simulink model "soft_radio"  (Simulink 6.4)
settings: Solver=FixedStepDiscrete  StartTime=0.0  StopTime=inf  RelTol=1e-3
StartFcn:
  | soft_radio_init
values from neighbouring files (symbols this model uses):
  atten1 = 0.1    [SDR (2).m]
  atten2 = 0.78    [SDR (2).m]
  atten3 = 0.25    [SDR (2).m]
  delay1 = 55    [SDR (2).m]
  delay2inc = 2    [SDR (2).m]
  delay3inc = 2    [SDR (2).m]
  Fmod = Fs/4    (= 24000)    [SDR (2).m]
  freq_off = 10    [SDR (2).m]
  Fs = 96000    [SDR (2).m]
  pnoise = 0.0005    [SDR (2).m]
  Ts = 1/Fs    (= 1.04166666667e-05)    [SDR (2).m]
undefined symbols (not defined in the file or in its folder): get, gray, j
libraries: simulink x29, dspbuff3 x27, dspsigops x18, dspsrcs4 x10, dspstat3 x7, dspindex x6, dsparch4 x5, commsink2 x4, dspmtrx3 x4, dspsnks4 x3, dspxfrm3 x2, commnoisgen2 x1
CloseFcn:
  | rtwprivate ssgencode ModelCloseRequest soft_radio
settings Model: LastModifiedBy=isa  ProdHWDeviceType=32-bit Generic Real Time Simulator
settings DataIOCC: ExternalInput=a  LoadExternalInput=on  SaveFormat=Structure  SaveOutput=off  SaveTime=off
settings OptimizationCC: InlineParams=on  InlineInvariantSignals=on  EnforceIntegerDowncast=off  StateBitsets=on  DataBitsets=on  UseTempVars=on  EfficientFloat2IntCast=on
settings DebuggingCC: SignalResolutionControl=UseLocalSettings  InheritedTsInSrcMsg=none  IntegerOverflowMsg=none  StrictBusMsg=ErrorLevel1
settings HardwareCC: ProdHWDeviceType=32-bit Generic Real Time Simulator  TargetHWDeviceType=32-bit Generic
settings RTWCC: GenCodeOnly=on  ProcessScript=grt_make_rtw_hook

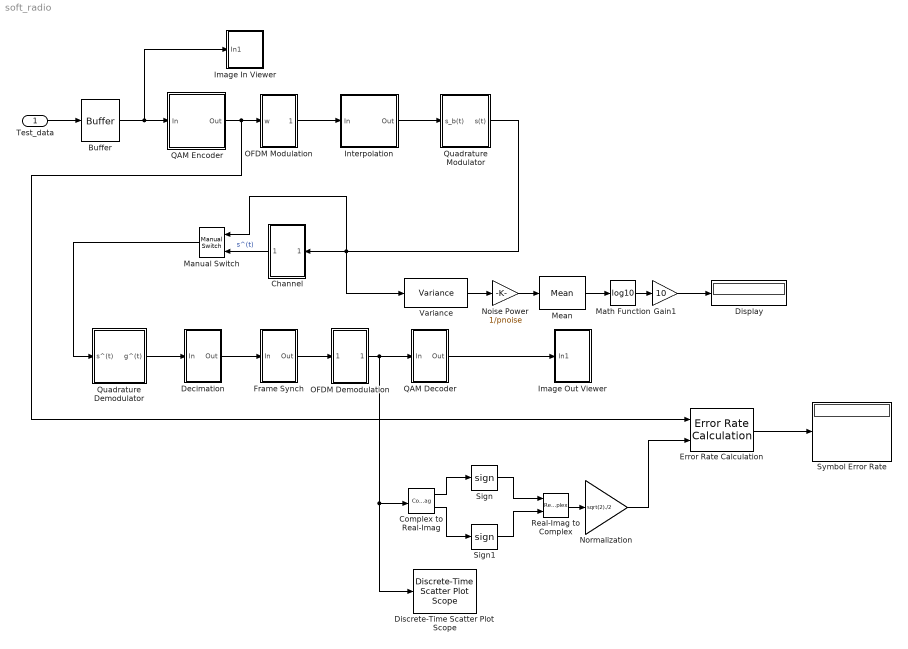
== system soft_radio ==
  Test_data : Inport  PortDimensions=1  SampleTime=1/(5*125)  DataType=uint8  Interpolate=off
  Buffer : dspbuff3/Buffer  N=256  V=0  ic=255
  Channel : Subsystem  Orientation=left
  Complex to Real-Imag : ComplexToRealImag
  Decimation : Subsystem
  Discrete-Time Scatter Plot Scope : commsink2/Discrete-Time Scatter Plot Scope  Tag=ScatterPlot  SystemSampleTime=-1  sampPerSymb=1  offsetEye=0  numTraces=40  numNewFrames=10  LineMarkers=.  LineColors=b  fading=on  render=on  AxisGrid=on  xMin=-1.87322652919263  xMax=1.91980304391689  yMin=-1.85318186191091  yMax=1.93984771119861  inphaseLabel=In-phase Amplitude  quadratureLabel=Quadrature Amplitude  openScopeAtSimStart=on  FrameNumber=off  FigPos=[360 138 560 560]  figTitle=Scatter Plot  numLinesMax=8  block_type_=scatter
  Display : Display
  Error Rate Calculation : commsink2/Error Rate Calculation  N=940  st_delay=0  cp_mode=Entire frame  subframe=[]  PMode=Port  WsName=ErrorVec  RsMode2=off  stop=off  numErr=1  maxBits=1
  Frame Synch : Subsystem
  Gain1 : Gain  Gain=10
  Image In Viewer : Subsystem
  Image Out Viewer : Subsystem
  "Interpolation " : Subsystem
  Manual Switch : simulink/Signal Routing/Manual Switch  Orientation=left  SystemSampleTime=-1  sw=1  action=0
  Math Function : Math  Operator=log10  SaturateOnIntegerOverflow=on
  Mean : dspstat3/Mean  DialogController=dspDDGCreate  DialogControllerArgs=DataTag10  run=on  reset_popup=None  roundingMode=Floor  overflowMode=off
  Noise Power : Gain  Gain=1/pnoise
  Normalization : Gain  Gain=sqrt(2)./2
  OFDM Demodulation : Subsystem
  OFDM Modulation : Subsystem
  QAM Decoder : Subsystem
  QAM Encoder : Subsystem
  Quadrature Demodulator : Subsystem
  Quadrature Modulator : Subsystem
  Real-Imag to Complex : RealImagToComplex
  Sign : Signum
  Sign1 : Signum
  Symbol Error Rate : Display
  Variance : dspstat3/Variance  DialogController=dspDDGCreate  DialogControllerArgs=DataTag15  run=off  reset_popup=None  roundingMode=Floor  overflowMode=off
  wires:
  Test_data/1 -> Buffer/1
  QAM Decoder/1(Out) -> Image Out Viewer/1(In1)
  Buffer/1 -> QAM Encoder/1(In), Image In Viewer/1(In1)
  OFDM Demodulation/1(w^) -> QAM Decoder/1(In), Discrete-Time Scatter Plot Scope/1, Complex to Real-Imag/1
  QAM Encoder/1(Out) -> OFDM Modulation/1(w), Error Rate Calculation/1
  OFDM Modulation/1(s_b(t)) -> "Interpolation "/1(In)
  "Interpolation "/1(Out) -> Quadrature Modulator/1(s_b(t))
  Quadrature Demodulator/1(g^(t)) -> Decimation/1(In)
  Decimation/1(Out) -> Frame Synch/1(In)
  Frame Synch/1(Out) -> OFDM Demodulation/1(g^(t))
  Quadrature Modulator/1(s(t)) -> Channel/1(s(t)), Manual Switch/1, Variance/1
  Channel/1(s^(t)) -> Manual Switch/2  "s^(t)"
  Manual Switch/1 -> Quadrature Demodulator/1(s^(t))
  Variance/1 -> Noise Power/1
  Noise Power/1 -> Mean/1
  Mean/1 -> Math Function/1
  Math Function/1 -> Gain1/1
  Gain1/1 -> Display/1
  Error Rate Calculation/1 -> Symbol Error Rate/1
  Complex to Real-Imag/1 -> Sign/1
  Complex to Real-Imag/2 -> Sign1/1
  Sign/1 -> Real-Imag to Complex/1
  Sign1/1 -> Real-Imag to Complex/2
  Real-Imag to Complex/1 -> Normalization/1
  Normalization/1 -> Error Rate Calculation/2

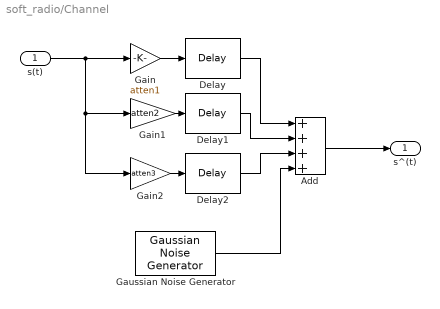
== system soft_radio/Channel ==
  s(t) : Inport
  Add : Sum  Inputs=++++  OutScaling=2^-10
  Delay : dspsigops/Delay  dly_unit=Samples  delay=delay1  ic_detail=off  dif_ic_for_ch=off  dif_ic_for_dly=off  ic=0  reset_popup=None
  Delay1 : dspsigops/Delay  dly_unit=Samples  delay=delay1+delay2inc  ic_detail=off  dif_ic_for_ch=off  dif_ic_for_dly=off  ic=0  reset_popup=None
  Delay2 : dspsigops/Delay  dly_unit=Samples  delay=delay1+delay3inc  ic_detail=off  dif_ic_for_ch=off  dif_ic_for_dly=off  ic=0  reset_popup=None
  Gain : Gain  Gain=atten1
  Gain1 : Gain  Gain=atten2
  Gain2 : Gain  Gain=atten3
  Gaussian Noise Generator : commnoisgen2/Gaussian Noise Generator  SystemSampleTime=-1  m=0  d=pnoise  s=noiseseed  Ts=-1  frameBased=on  sampPerFrame=96  orient=off  outDataType=double
  s^(t) : Outport
  wires:
  s(t)/1 -> Gain/1, Gain1/1, Gain2/1
  Gain/1 -> Delay/1
  Delay/1 -> Add/1
  Gain2/1 -> Delay2/1
  Gain1/1 -> Delay1/1
  Delay1/1 -> Add/2
  Delay2/1 -> Add/3
  Add/1 -> s^(t)/1
  Gaussian Noise Generator/1 -> Add/4

== system soft_radio/Decimation ==
  In : Inport
  Digital Filter Design : dsparch4/Digital Filter Design  SystemSampleTime=-1  mwdsp_browser_bugfix_var=off
  Digital Filter Design1 : dsparch4/Digital Filter Design  SystemSampleTime=-1  mwdsp_browser_bugfix_var=off
  Digital Filter Design2 : dsparch4/Digital Filter Design  SystemSampleTime=-1  mwdsp_browser_bugfix_var=off
  Downsample : dspsigops/Downsample  N=2  phase=0  ic=0  smode=Allow multirate  fmode=Maintain input frame size
  Downsample1 : dspsigops/Downsample  N=2  phase=0  ic=0  smode=Allow multirate  fmode=Maintain input frame size
  Downsample2 : dspsigops/Downsample  N=2  phase=0  ic=0  smode=Allow multirate  fmode=Maintain input frame size
  Out : Outport
  wires:
  Downsample/1 -> Out/1
  In/1 -> Digital Filter Design1/1
  Digital Filter Design1/1 -> Downsample1/1
  Downsample1/1 -> Digital Filter Design2/1
  Digital Filter Design2/1 -> Downsample2/1
  Downsample2/1 -> Digital Filter Design/1
  Digital Filter Design/1 -> Downsample/1

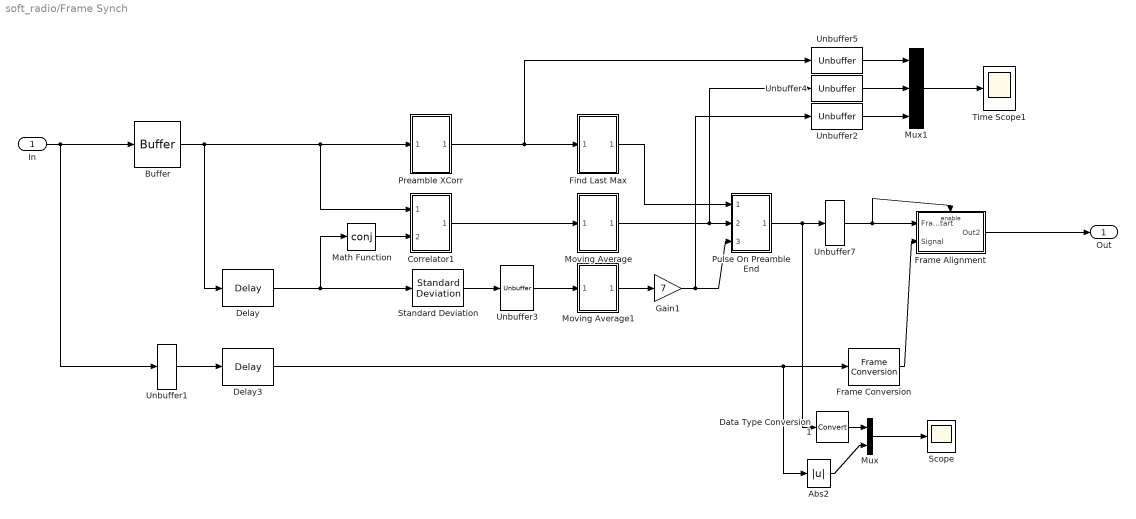
== system soft_radio/Frame Synch ==
  In : Inport
  Abs2 : Abs  SampleTime=-1  SaturateOnIntegerOverflow=off
  Buffer : dspbuff3/Buffer  N=161  V=160  ic=0
  Correlator1 : Subsystem
  Data Type Conversion1 : DataTypeConversion
  Delay : dspsigops/Delay  dly_unit=Frames  delay=161  ic_detail=off  dif_ic_for_ch=off  dif_ic_for_dly=off  ic=0  reset_popup=None
  Delay3 : dspsigops/Delay  dly_unit=Samples  delay=257-96  ic_detail=off  dif_ic_for_ch=off  dif_ic_for_dly=off  ic=0  reset_popup=None
  Find Last Max : Subsystem
  Frame Alignment : Subsystem  TreatAsAtomicUnit=on
  Frame Conversion : FrameConversion
  Gain1 : Gain  Gain=7
  Math Function : Math  Operator=conj  SaturateOnIntegerOverflow=on
  Moving Average : Subsystem
  Moving Average1 : Subsystem
  Mux : Mux  Inputs=2
  Mux1 : Mux  Inputs=3
  Preamble XCorr : Subsystem
  Pulse On Preamble End : Subsystem
  Scope : Scope
      settings: YMin=2.77556e-017  YMax=1  SaveName=frame_scope2  DataFormat=Array  MaxDataPoints=50000
  Standard Deviation : dspstat3/Standard Deviation  run=off  reset_popup=None
  Time Scope1 : Scope
      settings: TimeRange=3  YMin=5.55112e-017  YMax=2.1  DataFormat=Array  MaxDataPoints=50000
  Unbuffer{1..5,7} (6 alike) : dspbuff3/Unbuffer  ic=0
  Out : Outport
  wires:
  Buffer/1 -> Correlator1/1(In1), Preamble XCorr/1(In1), Delay/1
  In/1 -> Buffer/1, Unbuffer1/1
  Preamble XCorr/1(Out1) -> Find Last Max/1(In1), Unbuffer5/1
  Delay/1 -> Standard Deviation/1, Math Function/1
  Standard Deviation/1 -> Unbuffer3/1
  Unbuffer3/1 -> Moving Average1/1(In1)
  Moving Average/1(Out1) -> Pulse On Preamble End/2(In2), Unbuffer4/1
  Correlator1/1(Out1) -> Moving Average/1(In1)
  Moving Average1/1(Out1) -> Gain1/1
  Gain1/1 -> Pulse On Preamble End/3(In3), Unbuffer2/1
  Find Last Max/1(Out1) -> Pulse On Preamble End/1(In1)
  Pulse On Preamble End/1(Out1) -> Unbuffer7/1, Data Type Conversion1/1
  Delay3/1 -> Frame Conversion/1, Abs2/1
  Math Function/1 -> Correlator1/2(In2)
  Frame Conversion/1 -> Frame Alignment/2(Signal)
  Frame Alignment/1(Out2) -> Out/1
  Unbuffer7/1 -> Frame Alignment/1(Frame Start), Frame Alignment/Enable
  Abs2/1 -> Mux/2
  Mux/1 -> Scope/1
  Data Type Conversion1/1 -> Mux/1
  Mux1/1 -> Time Scope1/1
  Unbuffer2/1 -> Mux1/3
  Unbuffer4/1 -> Mux1/2
  Unbuffer5/1 -> Mux1/1
  Unbuffer1/1 -> Delay3/1

== system soft_radio/Image In Viewer ==
  In1 : Inport  Orientation=down
  Delay Line : dspbuff3/Delay Line  siz=256  ic=0  directfeed=off
  Matrix Viewer : dspsnks4/Matrix Viewer  DialogController=dspdialog.MatrixViewer  DialogControllerArgs=DataTag6  ImageParams=off  CMapStr=gray(256)  AxisColorbar=on  AxisParams=off  AxisOrigin=Upper left corner  XLabel=X-axis  YLabel=Y-axis  ZLabel=Z-axis  FigPos=get(0,'defaultfigureposition')  AxisZoom=off
      settings: YMin=0  YMax=255
  Transpose : dspmtrx3/Transpose  SystemSampleTime=-1  Hermitian=off  overflowFlag=on
  Transpose2 : dspmtrx3/Transpose  SystemSampleTime=-1  Hermitian=off  overflowFlag=on
  wires:
  In1/1 -> Transpose/1
  Transpose2/1 -> Matrix Viewer/1
  Delay Line/1 -> Transpose2/1
  Transpose/1 -> Delay Line/1

== system soft_radio/Image Out Viewer ==
  In1 : Inport  Orientation=down
  Delay Line : dspbuff3/Delay Line  siz=256  ic=0  directfeed=off
  Matrix Viewer : dspsnks4/Matrix Viewer  DialogController=dspdialog.MatrixViewer  DialogControllerArgs=DataTag7  ImageParams=off  CMapStr=gray(256)  AxisColorbar=on  AxisParams=off  AxisOrigin=Upper left corner  XLabel=X-axis  YLabel=Y-axis  ZLabel=Z-axis  FigPos=get(0,'defaultfigureposition')  AxisZoom=off
      settings: YMin=0  YMax=255
  Transpose : dspmtrx3/Transpose  SystemSampleTime=-1  Hermitian=off  overflowFlag=on
  Transpose2 : dspmtrx3/Transpose  SystemSampleTime=-1  Hermitian=off  overflowFlag=on
  wires:
  Transpose/1 -> Delay Line/1
  Delay Line/1 -> Transpose2/1
  Transpose2/1 -> Matrix Viewer/1
  In1/1 -> Transpose/1

== system soft_radio/Interpolation  ==
  In : Inport
  Initial Upsampling Filter : dsparch4/Digital Filter Design  SystemSampleTime=-1  mwdsp_browser_bugfix_var=off
  Second Upsample : dspsigops/Upsample  N=4  phase=0  ic=0  mode=Maintain input frame size
  Second Upsampling Filter : dsparch4/Digital Filter Design  SystemSampleTime=-1  mwdsp_browser_bugfix_var=off
  Upsample : dspsigops/Upsample  N=2  phase=0  ic=0  mode=Maintain input frame size
  Upsampling Amplitude Correction : Gain  Gain=8
  Out : Outport
  wires:
  Initial Upsampling Filter/1 -> Second Upsample/1
  Upsample/1 -> Initial Upsampling Filter/1
  Second Upsample/1 -> Second Upsampling Filter/1
  In/1 -> Upsample/1
  Second Upsampling Filter/1 -> Upsampling Amplitude Correction/1
  Upsampling Amplitude Correction/1 -> Out/1

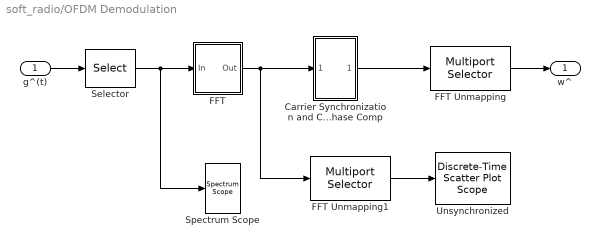
== system soft_radio/OFDM Demodulation ==
  g^(t) : Inport
  Carrier Synchronization and Channel Phase Comp : Subsystem
  FFT : Subsystem
  FFT Unmapping : dspindex/Multiport Selector  rowsOrCols=Rows  idxCellArray={[2, 3, 4, 5, 61, 62, 63, 64, 6, 7, 59, 60, 9, 10, 11, 12, 54, 55, 56, 57]}  idxErrMode=Clip Index
  FFT Unmapping1 : dspindex/Multiport Selector  rowsOrCols=Rows  idxCellArray={[2, 3, 4, 5, 61, 62, 63, 64, 6, 7, 59, 60, 9, 10, 11, 12, 54, 55, 56, 57]}  idxErrMode=Clip Index
  Selector : Selector  Elements=[25:88]  InputPortWidth=96
  Spectrum Scope : dspsnks4/Spectrum Scope  DialogController=dspdialog.SpectrumScope  DialogControllerArgs=DataTag13  SystemSampleTime=-1  ScopeProperties=on  Domain=Frequency  HorizSpan=1  UseBuffer=on  BufferSize=64  Overlap=0  inpFftLenInherit=off  FFTlength=128  numAvg=2  DisplayProperties=off  AxisGrid=on  Memory=off  FrameNumber=on  AxisLegend=off  AxisZoom=off  OpenScopeAtSimStart=on  OpenScopeImmediately=off  FigPos=get(0,'defaultfigureposition')  AxisProperties=off  XUnits=Hertz  XRange=[-Fs/2...Fs/2]  InheritXIncr=on  XIncr=1.0  XLabel=Samples  YUnits=dB  YLabel=Magnitude-squared, dB  LineProperties=off  wintypeSpecScope=Hann  RsSpecScope=50  betaSpecScope=5  winsampSpecScope=Periodic
      settings: YMin=-120.845322888998  YMax=-11.741242369477
  Unsynchronized : commsink2/Discrete-Time Scatter Plot Scope  Tag=ScatterPlot  SystemSampleTime=-1  sampPerSymb=1  offsetEye=0  numTraces=40  numNewFrames=10  LineMarkers=.  LineColors=b  fading=on  render=on  AxisGrid=on  xMin=-1.88995217282586  xMax=1.90933368918377  yMin=-1.88734763336516  yMax=1.91193822864447  inphaseLabel=In-phase Amplitude  quadratureLabel=Quadrature Amplitude  openScopeAtSimStart=on  FrameNumber=off  FigPos=[360 138 560 560]  figTitle=Scatter Plot  numLinesMax=8  block_type_=scatter
  w^ : Outport
  wires:
  g^(t)/1 -> Selector/1
  FFT Unmapping/1 -> w^/1
  Selector/1 -> FFT/1(In), Spectrum Scope/1
  FFT/1(Out) -> FFT Unmapping1/1, Carrier Synchronization and Channel Phase Comp/1(s(f))
  FFT Unmapping1/1 -> Unsynchronized/1
  Carrier Synchronization and Channel Phase Comp/1(s^(f)) -> FFT Unmapping/1

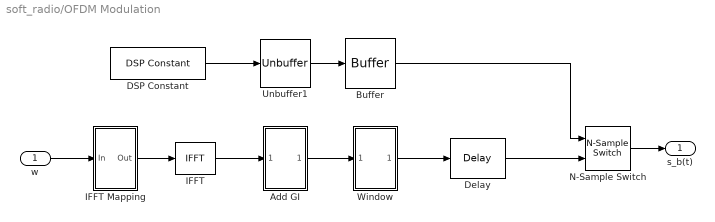
== system soft_radio/OFDM Modulation ==
  w : Inport
  Add GI : Subsystem
  Buffer : dspbuff3/Buffer  N=96  V=0  ic=0
  DSP Constant : dspsrcs4/DSP Constant  SystemSampleTime=-1  Value=preamble_whole'  SampleMode=Discrete  discreteOutput=Frame-based  continuousOutput=Sample-based  sampTime=-1  framePeriod=-1  dataType=Inherit from 'Constant value'  isSigned=on  wordLen=16  udDataType=sfix(16)  fracBitsMode=Best precision  numFracBits=15  InterpretAs1D=-inf  Ts=-inf  FramebasedOutput=-inf
  Delay : dspsigops/Delay  dly_unit=Frames  delay=39  ic_detail=off  dif_ic_for_ch=off  dif_ic_for_dly=off  ic=0  reset_popup=None
  IFFT : dspxfrm3/IFFT  DialogController=dspDDGCreate  DialogControllerArgs=DataTag14  CompMethod=Table lookup  TableOpt=Speed  BitRevOrder=off  cs_in=off  SkipNorm=off  mode=Complex  roundingMode=Floor  overflowMode=off
  IFFT Mapping : Subsystem
  N-Sample Switch : dspswit3/N-Sample Switch  SystemSampleTime=-1  N=39  reset=off  TriggerType=Rising edge  Ts=-1
  Unbuffer1 : dspbuff3/Unbuffer  ic=0
  Window : Subsystem
  s_b(t) : Outport
  wires:
  IFFT Mapping/1(Out) -> IFFT/1
  w/1 -> IFFT Mapping/1(In)
  IFFT/1 -> Add GI/1(In1)
  Add GI/1(Out1) -> Window/1(In1)
  Window/1(Out1) -> Delay/1
  N-Sample Switch/1 -> s_b(t)/1
  Buffer/1 -> N-Sample Switch/1
  DSP Constant/1 -> Unbuffer1/1
  Unbuffer1/1 -> Buffer/1
  Delay/1 -> N-Sample Switch/2

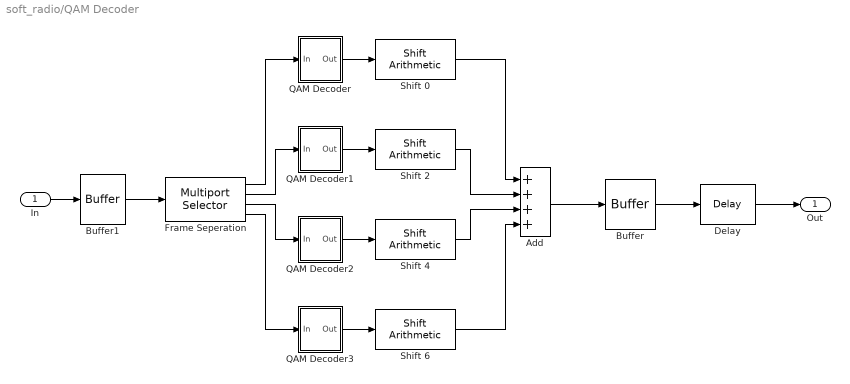
== system soft_radio/QAM Decoder ==
  In : Inport
  Add : Sum  Inputs=++++  OutScaling=2^-10
  Buffer : dspbuff3/Buffer  N=256  V=0  ic=0
  Buffer1 : dspbuff3/Buffer  N=4  V=0  ic=0
  Delay : dspsigops/Delay  dly_unit=Samples  delay=11  ic_detail=off  dif_ic_for_ch=off  dif_ic_for_dly=off  ic=0  reset_popup=None
  Frame Seperation : dspindex/Multiport Selector  rowsOrCols=Rows  idxCellArray={1,2,3,4}  idxErrMode=Clip Index
  QAM Decoder : Subsystem
  QAM Decoder1 : Subsystem
  QAM Decoder2 : Subsystem
  QAM Decoder3 : Subsystem
  Shift 0 : simulink/Logic and Bit Operations/Shift Arithmetic  SystemSampleTime=-1  nBitShiftRight=0  nBinPtShiftRight=0
  Shift 2 : simulink/Logic and Bit Operations/Shift Arithmetic  SystemSampleTime=-1  nBitShiftRight=-2  nBinPtShiftRight=0
  Shift 4 : simulink/Logic and Bit Operations/Shift Arithmetic  SystemSampleTime=-1  nBitShiftRight=-4  nBinPtShiftRight=0
  Shift 6 : simulink/Logic and Bit Operations/Shift Arithmetic  SystemSampleTime=-1  nBitShiftRight=-6  nBinPtShiftRight=0
  Out : Outport
  wires:
  Frame Seperation/1 -> QAM Decoder/1(In)
  QAM Decoder/1(Out) -> Shift 0/1
  Frame Seperation/2 -> QAM Decoder1/1(In)
  Frame Seperation/3 -> QAM Decoder2/1(In)
  Frame Seperation/4 -> QAM Decoder3/1(In)
  QAM Decoder1/1(Out) -> Shift 2/1
  QAM Decoder2/1(Out) -> Shift 4/1
  QAM Decoder3/1(Out) -> Shift 6/1
  Shift 0/1 -> Add/1
  Shift 2/1 -> Add/2
  Shift 4/1 -> Add/3
  Shift 6/1 -> Add/4
  Add/1 -> Buffer/1
  In/1 -> Buffer1/1
  Buffer/1 -> Delay/1
  Delay/1 -> Out/1
  Buffer1/1 -> Frame Seperation/1

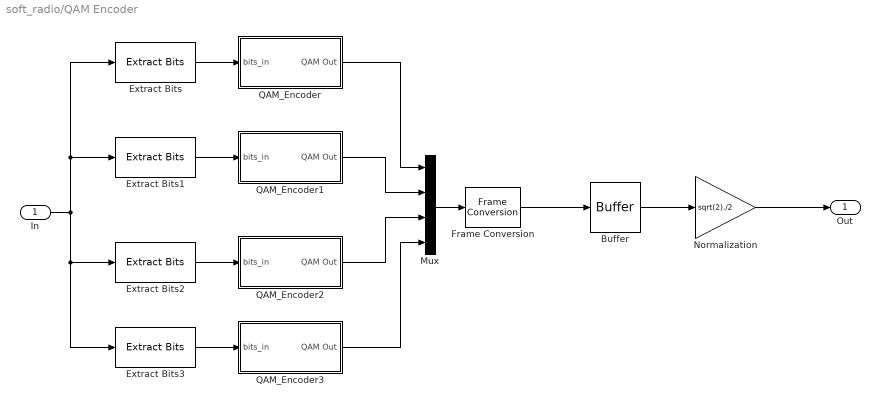
== system soft_radio/QAM Encoder ==
  In : Inport
  Buffer : dspbuff3/Buffer  N=20  V=0  ic=-1-j
  Extract Bits : simulink/Logic and Bit Operations/Extract Bits  SystemSampleTime=-1  bitsToExtract=Range of bits  numBits=2  bitIdxRange=[0 1]  outScalingMode=Treat bit field as an integer
  Extract Bits1 : simulink/Logic and Bit Operations/Extract Bits  SystemSampleTime=-1  bitsToExtract=Range of bits  numBits=2  bitIdxRange=[2 3]  outScalingMode=Treat bit field as an integer
  Extract Bits2 : simulink/Logic and Bit Operations/Extract Bits  SystemSampleTime=-1  bitsToExtract=Range of bits  numBits=2  bitIdxRange=[4 5]  outScalingMode=Treat bit field as an integer
  Extract Bits3 : simulink/Logic and Bit Operations/Extract Bits  SystemSampleTime=-1  bitsToExtract=Range of bits  numBits=2  bitIdxRange=[6 7]  outScalingMode=Treat bit field as an integer
  Frame Conversion : FrameConversion
  Mux : Mux
  Normalization : Gain  Gain=sqrt(2)./2
  QAM_Encoder : Subsystem
  QAM_Encoder1 : Subsystem
  QAM_Encoder2 : Subsystem
  QAM_Encoder3 : Subsystem
  Out : Outport
  wires:
  In/1 -> Extract Bits1/1, Extract Bits/1, Extract Bits2/1, Extract Bits3/1
  Extract Bits/1 -> QAM_Encoder/1(bits_in)
  Extract Bits1/1 -> QAM_Encoder1/1(bits_in)
  Extract Bits2/1 -> QAM_Encoder2/1(bits_in)
  Extract Bits3/1 -> QAM_Encoder3/1(bits_in)
  QAM_Encoder/1(QAM Out) -> Mux/1
  QAM_Encoder1/1(QAM Out) -> Mux/2
  QAM_Encoder2/1(QAM Out) -> Mux/3
  QAM_Encoder3/1(QAM Out) -> Mux/4
  Mux/1 -> Frame Conversion/1
  Frame Conversion/1 -> Buffer/1
  Buffer/1 -> Normalization/1
  Normalization/1 -> Out/1

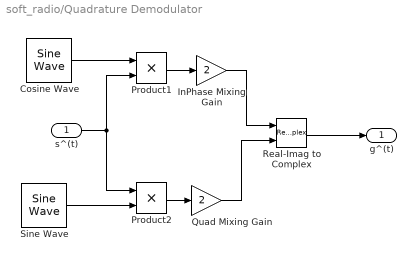
== system soft_radio/Quadrature Demodulator ==
  s^(t) : Inport
  Cosine Wave : dspsrcs4/Sine Wave  Amplitude=1  Frequency=Fmod+freq_off  Phase=pi/2  SampleMode=Discrete  OutComplex=Real  CompMethod=Trigonometric fcn  TableSize=Speed  SampleTime=Ts  SamplesPerFrame=96  dataType=double  wordLen=16  udDataType=sfix(16)  fracBitsMode=Best precision  numFracBits=15  ResetState=Restart at time zero
  InPhase Mixing Gain : Gain  Gain=2
  Product1 : Product  RndMeth=Zero
  Product2 : Product  RndMeth=Zero
  Quad Mixing Gain : Gain  Gain=2
  Real-Imag to Complex : RealImagToComplex
  Sine Wave : dspsrcs4/Sine Wave  Amplitude=1  Frequency=Fmod+freq_off  Phase=0  SampleMode=Discrete  OutComplex=Real  CompMethod=Trigonometric fcn  TableSize=Speed  SampleTime=Ts  SamplesPerFrame=96  dataType=double  wordLen=16  udDataType=sfix(16)  fracBitsMode=Best precision  numFracBits=15  ResetState=Restart at time zero
  g^(t) : Outport
  wires:
  s^(t)/1 -> Product1/2, Product2/1
  Cosine Wave/1 -> Product1/1
  Sine Wave/1 -> Product2/2
  Product1/1 -> InPhase Mixing Gain/1
  Product2/1 -> Quad Mixing Gain/1
  Quad Mixing Gain/1 -> Real-Imag to Complex/2
  InPhase Mixing Gain/1 -> Real-Imag to Complex/1
  Real-Imag to Complex/1 -> g^(t)/1

== system soft_radio/Quadrature Modulator ==
  s_b(t) : Inport
  Add : Sum  OutScaling=2^-10
  Complex to Real-Imag : ComplexToRealImag
  Cosine Wave : dspsrcs4/Sine Wave  Amplitude=1  Frequency=Fmod  Phase=pi/2  SampleMode=Discrete  OutComplex=Real  CompMethod=Trigonometric fcn  TableSize=Speed  SampleTime=Ts  SamplesPerFrame=96  dataType=double  wordLen=16  udDataType=sfix(16)  fracBitsMode=Best precision  numFracBits=15  ResetState=Restart at time zero
  Product : Product  RndMeth=Zero
  Product2 : Product  RndMeth=Zero
  Sine Wave : dspsrcs4/Sine Wave  Amplitude=1  Frequency=Fmod  Phase=0  SampleMode=Discrete  OutComplex=Real  CompMethod=Trigonometric fcn  TableSize=Speed  SampleTime=Ts  SamplesPerFrame=96  dataType=double  wordLen=16  udDataType=sfix(16)  fracBitsMode=Best precision  numFracBits=15  ResetState=Restart at time zero
  s(t) : Outport
  wires:
  Add/1 -> s(t)/1
  Product/1 -> Add/1
  Product2/1 -> Add/2
  Cosine Wave/1 -> Product/1
  s_b(t)/1 -> Complex to Real-Imag/1
  Complex to Real-Imag/2 -> Product2/1
  Complex to Real-Imag/1 -> Product/2
  Sine Wave/1 -> Product2/2

== system soft_radio/Frame Synch/Correlator1 ==
  In1 : Inport
  In2 : Inport  Port=2
  Abs2 : Abs  SampleTime=-1  SaturateOnIntegerOverflow=off
  Product1 : Product  RndMeth=Zero
  Sum of Elements1 : Sum  Inputs=+  OutScaling=2^-10
  Out1 : Outport
  wires:
  Product1/1 -> Sum of Elements1/1
  Sum of Elements1/1 -> Abs2/1
  In1/1 -> Product1/1
  In2/1 -> Product1/2
  Abs2/1 -> Out1/1

== system soft_radio/Frame Synch/Find Last Max ==
  In1 : Inport
  Compare To Constant : simulink/Logic and Bit Operations/Compare To Constant  SystemSampleTime=-1  relop===  const=64  LogicOutDataTypeMode=uint8  ZeroCross=off
  Delay Line1 : dspbuff3/Delay Line  siz=64  ic=0  directfeed=off
  Maximum : dspstat3/Maximum  DialogController=dspDDGCreate  DialogControllerArgs=DataTag3  fcn=Index  reset=None  roundingMode=Floor  overflowMode=off
  Out1 : Outport
  wires:
  Delay Line1/1 -> Maximum/1
  Maximum/1 -> Compare To Constant/1
  In1/1 -> Delay Line1/1
  Compare To Constant/1 -> Out1/1

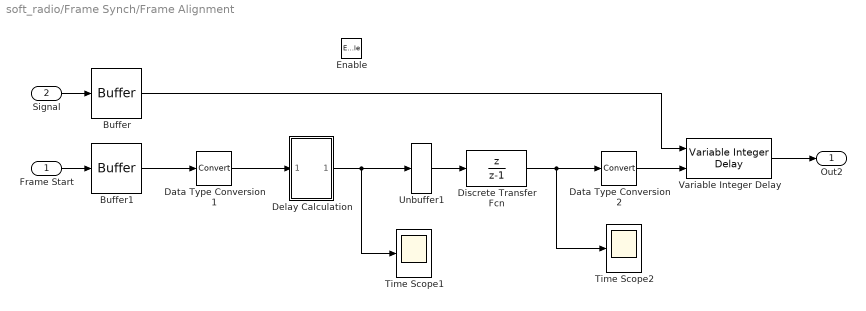
== system soft_radio/Frame Synch/Frame Alignment ==
  Frame Start : Inport
  Signal : Inport  Port=2
      settings: SignalType=complex
  Enable : EnablePort  StatesWhenEnabling=reset
  Buffer : dspbuff3/Buffer  N=96  V=0  ic=0
  Buffer1 : dspbuff3/Buffer  N=96  V=0  ic=0
  Data Type Conversion1 : DataTypeConversion
  Data Type Conversion2 : DataTypeConversion
  Delay Calculation : Subsystem
  Discrete Transfer Fcn : DiscreteTransferFcn  Numerator=[1 0]  Denominator=[1 -1]  SampleTime=-1
  Time Scope1 : Scope
      settings: YMax=10  SaveName=ScopeData3  DataFormat=Structure
  Time Scope2 : Scope
      settings: YMin=0  YMax=70  SaveName=ScopeData2  DataFormat=Structure
  Unbuffer1 : dspbuff3/Unbuffer  ic=0
  Variable Integer Delay : dspsigops/Variable Integer Delay  dmax=100  ic=0
  Out2 : Outport  InitialOutput=[-2*ones(64,0)]
  wires:
  Signal/1 -> Buffer/1
  Frame Start/1 -> Buffer1/1
  Buffer1/1 -> Data Type Conversion1/1
  Delay Calculation/1(Out1) -> Time Scope1/1, Unbuffer1/1
  Variable Integer Delay/1 -> Out2/1
  Discrete Transfer Fcn/1 -> Data Type Conversion2/1, Time Scope2/1
  Data Type Conversion1/1 -> Delay Calculation/1(In1)
  Buffer/1 -> Variable Integer Delay/1
  Unbuffer1/1 -> Discrete Transfer Fcn/1
  Data Type Conversion2/1 -> Variable Integer Delay/2

== system soft_radio/Frame Synch/Moving Average ==
  In1 : Inport
  Delay Line : dspbuff3/Delay Line  siz=128  ic=0  directfeed=off
  Mean : dspstat3/Mean  DialogController=dspDDGCreate  DialogControllerArgs=DataTag4  run=off  reset_popup=None  roundingMode=Floor  overflowMode=off
  Out1 : Outport
  wires:
  Delay Line/1 -> Mean/1
  In1/1 -> Delay Line/1
  Mean/1 -> Out1/1

== system soft_radio/Frame Synch/Moving Average1 ==
  In1 : Inport
  Delay Line2 : dspbuff3/Delay Line  siz=64  ic=0  directfeed=off
  Mean1 : dspstat3/Mean  DialogController=dspDDGCreate  DialogControllerArgs=DataTag5  run=off  reset_popup=None  roundingMode=Floor  overflowMode=off
  Out1 : Outport
  wires:
  Delay Line2/1 -> Mean1/1
  In1/1 -> Delay Line2/1
  Mean1/1 -> Out1/1

== system soft_radio/Frame Synch/Preamble XCorr ==
  In1 : Inport  Orientation=down
  Correlator : Subsystem
  Math Function1 : Math  Operator=conj  SaturateOnIntegerOverflow=on
  Short Sequence : dspsrcs4/DSP Constant  SystemSampleTime=-1  Value=short_seq_r'  SampleMode=Discrete  discreteOutput=Frame-based  continuousOutput=Sample-based  sampTime=1/(96e3)  framePeriod=-1  dataType=Inherit from 'Constant value'  isSigned=on  wordLen=16  udDataType=sfix(16)  fracBitsMode=Best precision  numFracBits=15  InterpretAs1D=-inf  Ts=-inf  FramebasedOutput=-inf
  Out1 : Outport
  wires:
  Short Sequence/1 -> Math Function1/1
  Math Function1/1 -> Correlator/1(In1)
  In1/1 -> Correlator/2(In2)
  Correlator/1(Out1) -> Out1/1

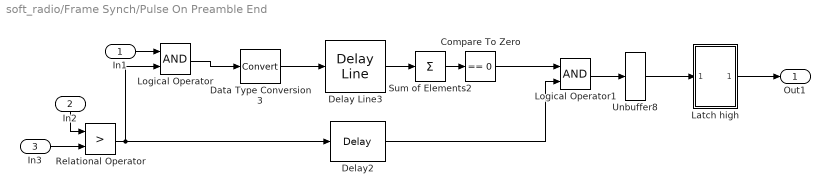
== system soft_radio/Frame Synch/Pulse On Preamble End ==
  In1 : Inport
  In2 : Inport  Orientation=down  Port=2
  In3 : Inport  Port=3
  Compare To Zero : simulink/Logic and Bit Operations/Compare To Zero  SystemSampleTime=-1  relop===  LogicOutDataTypeMode=uint8  ZeroCross=off
  Data Type Conversion3 : DataTypeConversion
  Delay Line3 : dspbuff3/Delay Line  siz=256  ic=0  directfeed=off
  Delay2 : dspsigops/Delay  dly_unit=Samples  delay=256  ic_detail=off  dif_ic_for_ch=off  dif_ic_for_dly=off  ic=0  reset_popup=None
  Latch high : Subsystem
  Logical Operator : Logic  AllPortsSameDT=off  OutDataTypeMode=Boolean
  Logical Operator1 : Logic  AllPortsSameDT=off  OutDataTypeMode=Boolean
  Relational Operator : RelationalOperator  Operator=>  LogicOutDataTypeMode=Boolean
  Sum of Elements2 : Sum  Inputs=+  OutScaling=2^-10
  Unbuffer8 : dspbuff3/Unbuffer  ic=0
  Out1 : Outport
  wires:
  Relational Operator/1 -> Logical Operator/2, Delay2/1
  Logical Operator/1 -> Data Type Conversion3/1
  Data Type Conversion3/1 -> Delay Line3/1
  Delay Line3/1 -> Sum of Elements2/1
  Sum of Elements2/1 -> Compare To Zero/1
  Compare To Zero/1 -> Logical Operator1/1
  Delay2/1 -> Logical Operator1/2
  In2/1 -> Relational Operator/1
  In3/1 -> Relational Operator/2
  In1/1 -> Logical Operator/1
  Logical Operator1/1 -> Unbuffer8/1
  Latch high/1(Out1) -> Out1/1
  Unbuffer8/1 -> Latch high/1(In1)

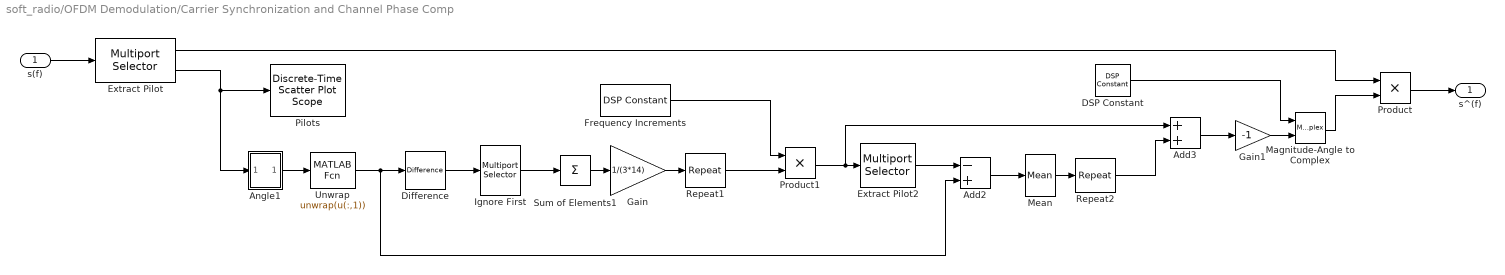
== system soft_radio/OFDM Demodulation/Carrier Synchronization and Channel Phase Comp ==
  s(f) : Inport
  Add2 : Sum  Inputs=-+  OutScaling=2^-10
  Add3 : Sum  OutScaling=2^-10
  Angle1 : Subsystem
  DSP Constant : dspsrcs4/DSP Constant  SystemSampleTime=-1  Value=1  SampleMode=Discrete  discreteOutput=Sample-based  continuousOutput=Sample-based  sampTime=-1  framePeriod=2  dataType=Inherit from 'Constant value'  isSigned=on  wordLen=16  udDataType=sfix(16)  fracBitsMode=Best precision  numFracBits=15  InterpretAs1D=-inf  Ts=-inf  FramebasedOutput=-inf
  Difference : simulink/Discrete/Difference  SystemSampleTime=-1  ICPrevInput=0.0  OutDataType=sfix(16)  OutScaling=2^-10  DoSatur=off
  Extract Pilot : dspindex/Multiport Selector  rowsOrCols=Rows  idxCellArray={[1:64],[44, 58, 8, 22]}  idxErrMode=Clip Index
  Extract Pilot2 : dspindex/Multiport Selector  rowsOrCols=Rows  idxCellArray={[44, 58, 8, 22]}  idxErrMode=Clip Index
  Frequency Increments : dspsrcs4/DSP Constant  SystemSampleTime=-1  Value=[32:63 0:31]'  SampleMode=Discrete  discreteOutput=Sample-based  continuousOutput=Sample-based  sampTime=-1  framePeriod=2  dataType=Inherit from 'Constant value'  isSigned=on  wordLen=16  udDataType=sfix(16)  fracBitsMode=Best precision  numFracBits=15  InterpretAs1D=-inf  Ts=-inf  FramebasedOutput=-inf
  Gain : Gain  Gain=1/(3*14)
  Gain1 : Gain  Gain=-1
  Ignore First : dspindex/Multiport Selector  rowsOrCols=Rows  idxCellArray={[2:4]}  idxErrMode=Clip Index
  Magnitude-Angle to Complex : MagnitudeAngleToComplex
  Mean : dspstat3/Mean  DialogController=dspDDGCreate  DialogControllerArgs=DataTag11  run=off  reset_popup=None  roundingMode=Floor  overflowMode=off
  Pilots : commsink2/Discrete-Time Scatter Plot Scope  Tag=ScatterPlot  SystemSampleTime=-1  sampPerSymb=1  offsetEye=0  numTraces=40  numNewFrames=10  LineMarkers=.  LineColors=b  fading=on  render=on  AxisGrid=on  xMin=-1.3  xMax=1.3  yMin=-1.3  yMax=1.3  inphaseLabel=In-phase Amplitude  quadratureLabel=Quadrature Amplitude  openScopeAtSimStart=off  FrameNumber=off  FigPos=[360 138 560 560]  figTitle=Scatter Plot  numLinesMax=8  block_type_=scatter
  Product : Product  RndMeth=Zero
  Product1 : Product  RndMeth=Zero
  Repeat1 : dspsigops/Repeat  N=64  ic=0  mode=Maintain input frame rate
  Repeat2 : dspsigops/Repeat  N=64  ic=0  mode=Maintain input frame rate
  Sum of Elements1 : Sum  Inputs=+  OutScaling=2^-10
  Unwrap : MATLABFcn  MATLABFcn=unwrap(u(:,1))  Output1D=off
  s^(f) : Outport
  wires:
  DSP Constant/1 -> Magnitude-Angle to Complex/1
  Magnitude-Angle to Complex/1 -> Product/2
  Product/1 -> s^(f)/1
  Extract Pilot/2 -> Angle1/1(In), Pilots/1
  s(f)/1 -> Extract Pilot/1
  Extract Pilot/1 -> Product/1
  Difference/1 -> Ignore First/1
  Sum of Elements1/1 -> Gain/1
  Gain/1 -> Repeat1/1
  Angle1/1(Out) -> Unwrap/1
  Unwrap/1 -> Difference/1, Add2/2
  Ignore First/1 -> Sum of Elements1/1
  Frequency Increments/1 -> Product1/1
  Repeat1/1 -> Product1/2
  Product1/1 -> Extract Pilot2/1, Add3/1
  Extract Pilot2/1 -> Add2/1
  Add2/1 -> Mean/1
  Mean/1 -> Repeat2/1
  Repeat2/1 -> Add3/2
  Add3/1 -> Gain1/1
  Gain1/1 -> Magnitude-Angle to Complex/2

== system soft_radio/OFDM Demodulation/FFT ==
  In : Inport
  FFT : dspxfrm3/FFT  DialogController=dspDDGCreate  DialogControllerArgs=DataTag12  CompMethod=Table lookup  TableOpt=Speed  BitRevOrder=off  SkipNorm=on  roundingMode=Floor  overflowMode=off
  Frame Conversion : FrameConversion
  Out : Outport
  wires:
  In/1 -> FFT/1
  Frame Conversion/1 -> Out/1
  FFT/1 -> Frame Conversion/1

== system soft_radio/OFDM Modulation/Add GI ==
  In1 : Inport
  Selector : Selector  Elements=[41:48 49:64 1:64 1:8]  InputPortWidth=96
  Zero Pad : dspsigops/Zero Pad  padSigAt=End  zpadAlong=Columns  padNumOutRowsSpecMethod=User-specified  numOutRows=96  padNumOutColsSpecMethod=User-specified  numOutCols=1  trunc_flag=None  isVarDimsMode=off
  Out1 : Outport
  wires:
  Zero Pad/1 -> Selector/1
  In1/1 -> Zero Pad/1
  Selector/1 -> Out1/1

== system soft_radio/OFDM Modulation/IFFT Mapping ==
  In : Inport
  Add : Sum  OutScaling=2^-10
  Selector : Selector  Elements=[64 1 2 3 4 9 10 63 13 14 15 16 21:61 17 18 19 20 62 11 12 5 6 7 8]  InputPortWidth=64
  Zero Pad : dspsigops/Zero Pad  padSigAt=End  zpadAlong=Columns  padNumOutRowsSpecMethod=User-specified  numOutRows=64  padNumOutColsSpecMethod=User-specified  numOutCols=1  trunc_flag=None  isVarDimsMode=off
  pilots : dspsrcs4/DSP Constant  SystemSampleTime=-1  Value=vertcat(zeros(7,1), 1, zeros(13,1), 1, zeros(21,1), 1, zeros(13,1), 1, zeros(6,1))  SampleMode=Discrete  discreteOutput=Sample-based  continuousOutput=Sample-based  sampTime=1/125  framePeriod=2  dataType=Inherit from 'Constant value'  isSigned=on  wordLen=16  udDataType=sfix(16)  fracBitsMode=Best precision  numFracBits=15  InterpretAs1D=-inf  Ts=-inf  FramebasedOutput=-inf
  Out : Outport
  wires:
  In/1 -> Zero Pad/1
  Zero Pad/1 -> Selector/1
  Selector/1 -> Add/1
  Add/1 -> Out/1
  pilots/1 -> Add/2

== system soft_radio/OFDM Modulation/Window ==
  In1 : Inport
  DSP Constant : dspsrcs4/DSP Constant  SystemSampleTime=-1  Value=w'  SampleMode=Discrete  discreteOutput=Sample-based  continuousOutput=Sample-based  sampTime=-1  framePeriod=2  dataType=Inherit from 'Constant value'  isSigned=on  wordLen=16  udDataType=sfix(16)  fracBitsMode=Best precision  numFracBits=15  InterpretAs1D=-inf  Ts=-inf  FramebasedOutput=-inf
  Product : Product  RndMeth=Zero
  Out1 : Outport
  wires:
  DSP Constant/1 -> Product/2
  In1/1 -> Product/1
  Product/1 -> Out1/1

== system soft_radio/QAM Decoder/QAM Decoder ==
  In : Inport
  Add : Sum  OutScaling=2^-10
  Compare To Zero : simulink/Logic and Bit Operations/Compare To Zero  SystemSampleTime=-1  relop=>  LogicOutDataTypeMode=uint8  ZeroCross=off
  Compare To Zero1 : simulink/Logic and Bit Operations/Compare To Zero  SystemSampleTime=-1  relop=>  LogicOutDataTypeMode=uint8  ZeroCross=off
  Complex to Real-Imag : ComplexToRealImag
  Shift By 1 : simulink/Logic and Bit Operations/Shift Arithmetic  SystemSampleTime=-1  nBitShiftRight=-1  nBinPtShiftRight=0
  Out : Outport
  wires:
  Complex to Real-Imag/1 -> Compare To Zero/1
  Complex to Real-Imag/2 -> Compare To Zero1/1
  Add/1 -> Out/1
  In/1 -> Complex to Real-Imag/1
  Compare To Zero/1 -> Shift By 1/1
  Shift By 1/1 -> Add/1
  Compare To Zero1/1 -> Add/2

== system soft_radio/QAM Decoder/QAM Decoder1 ==
  In : Inport
  Add : Sum  OutScaling=2^-10
  Compare To Zero : simulink/Logic and Bit Operations/Compare To Zero  SystemSampleTime=-1  relop=>  LogicOutDataTypeMode=uint8  ZeroCross=off
  Compare To Zero1 : simulink/Logic and Bit Operations/Compare To Zero  SystemSampleTime=-1  relop=>  LogicOutDataTypeMode=uint8  ZeroCross=off
  Complex to Real-Imag : ComplexToRealImag
  Shift By 1 : simulink/Logic and Bit Operations/Shift Arithmetic  SystemSampleTime=-1  nBitShiftRight=-1  nBinPtShiftRight=0
  Out : Outport
  wires:
  Compare To Zero1/1 -> Add/2
  Shift By 1/1 -> Add/1
  Compare To Zero/1 -> Shift By 1/1
  In/1 -> Complex to Real-Imag/1
  Add/1 -> Out/1
  Complex to Real-Imag/2 -> Compare To Zero1/1
  Complex to Real-Imag/1 -> Compare To Zero/1

== system soft_radio/QAM Decoder/QAM Decoder2 ==
  In : Inport
  Add : Sum  OutScaling=2^-10
  Compare To Zero : simulink/Logic and Bit Operations/Compare To Zero  SystemSampleTime=-1  relop=>  LogicOutDataTypeMode=uint8  ZeroCross=off
  Compare To Zero1 : simulink/Logic and Bit Operations/Compare To Zero  SystemSampleTime=-1  relop=>  LogicOutDataTypeMode=uint8  ZeroCross=off
  Complex to Real-Imag : ComplexToRealImag
  Shift By 1 : simulink/Logic and Bit Operations/Shift Arithmetic  SystemSampleTime=-1  nBitShiftRight=-1  nBinPtShiftRight=0
  Out : Outport
  wires:
  Complex to Real-Imag/1 -> Compare To Zero/1
  Complex to Real-Imag/2 -> Compare To Zero1/1
  Add/1 -> Out/1
  In/1 -> Complex to Real-Imag/1
  Compare To Zero/1 -> Shift By 1/1
  Shift By 1/1 -> Add/1
  Compare To Zero1/1 -> Add/2

== system soft_radio/QAM Decoder/QAM Decoder3 ==
  In : Inport
  Add : Sum  OutScaling=2^-10
  Compare To Zero : simulink/Logic and Bit Operations/Compare To Zero  SystemSampleTime=-1  relop=>  LogicOutDataTypeMode=uint8  ZeroCross=off
  Compare To Zero1 : simulink/Logic and Bit Operations/Compare To Zero  SystemSampleTime=-1  relop=>  LogicOutDataTypeMode=uint8  ZeroCross=off
  Complex to Real-Imag : ComplexToRealImag
  Shift By 1 : simulink/Logic and Bit Operations/Shift Arithmetic  SystemSampleTime=-1  nBitShiftRight=-1  nBinPtShiftRight=0
  Out : Outport
  wires:
  Compare To Zero1/1 -> Add/2
  Shift By 1/1 -> Add/1
  Compare To Zero/1 -> Shift By 1/1
  In/1 -> Complex to Real-Imag/1
  Add/1 -> Out/1
  Complex to Real-Imag/2 -> Compare To Zero1/1
  Complex to Real-Imag/1 -> Compare To Zero/1

== system soft_radio/QAM Encoder/QAM_Encoder ==
  bits_in : Inport
  Data Type Conversion : DataTypeConversion  OutDataTypeMode=uint8
  Direct Lookup Table (n-D) : simulink/Lookup Tables/Direct Lookup Table (n-D)  maskTabDims=1  explicitNumDims=1  outDims=Element  tabIsInput=off  mxTable=[-1-j,-1+j,1-j,1+j]  clipFlag=Warning
  Unbuffer : dspbuff3/Unbuffer  ic=0
  QAM Out : Outport
  wires:
  bits_in/1 -> Data Type Conversion/1
  Direct Lookup Table (n-D)/1 -> QAM Out/1
  Unbuffer/1 -> Direct Lookup Table (n-D)/1
  Data Type Conversion/1 -> Unbuffer/1

== system soft_radio/QAM Encoder/QAM_Encoder1 ==
  bits_in : Inport
  Data Type Conversion : DataTypeConversion  OutDataTypeMode=uint8
  Direct Lookup Table (n-D) : simulink/Lookup Tables/Direct Lookup Table (n-D)  maskTabDims=1  explicitNumDims=1  outDims=Element  tabIsInput=off  mxTable=[-1-j,-1+j,1-j,1+j]  clipFlag=Warning
  Unbuffer : dspbuff3/Unbuffer  ic=0
  QAM Out : Outport
  wires:
  Data Type Conversion/1 -> Unbuffer/1
  Unbuffer/1 -> Direct Lookup Table (n-D)/1
  Direct Lookup Table (n-D)/1 -> QAM Out/1
  bits_in/1 -> Data Type Conversion/1

== system soft_radio/QAM Encoder/QAM_Encoder2 ==
  bits_in : Inport
  Data Type Conversion : DataTypeConversion  OutDataTypeMode=uint8
  Direct Lookup Table (n-D) : simulink/Lookup Tables/Direct Lookup Table (n-D)  maskTabDims=1  explicitNumDims=1  outDims=Element  tabIsInput=off  mxTable=[-1-j,-1+j,1-j,1+j]  clipFlag=Warning
  Unbuffer : dspbuff3/Unbuffer  ic=0
  QAM Out : Outport
  wires:
  bits_in/1 -> Data Type Conversion/1
  Direct Lookup Table (n-D)/1 -> QAM Out/1
  Unbuffer/1 -> Direct Lookup Table (n-D)/1
  Data Type Conversion/1 -> Unbuffer/1

== system soft_radio/QAM Encoder/QAM_Encoder3 ==
  bits_in : Inport
  Data Type Conversion : DataTypeConversion  OutDataTypeMode=uint8
  Direct Lookup Table (n-D) : simulink/Lookup Tables/Direct Lookup Table (n-D)  maskTabDims=1  explicitNumDims=1  outDims=Element  tabIsInput=off  mxTable=[-1-j,-1+j,1-j,1+j]  clipFlag=Warning
  Unbuffer : dspbuff3/Unbuffer  ic=0
  QAM Out : Outport
  wires:
  Data Type Conversion/1 -> Unbuffer/1
  Unbuffer/1 -> Direct Lookup Table (n-D)/1
  Direct Lookup Table (n-D)/1 -> QAM Out/1
  bits_in/1 -> Data Type Conversion/1

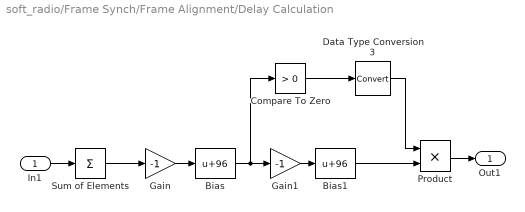
== system soft_radio/Frame Synch/Frame Alignment/Delay Calculation ==
  In1 : Inport
  Bias : Bias  Bias=96
  Bias1 : Bias  Bias=96
  Compare To Zero : simulink/Logic and Bit Operations/Compare To Zero  SystemSampleTime=-1  relop=>  LogicOutDataTypeMode=uint8  ZeroCross=off
  Data Type Conversion3 : DataTypeConversion
  Gain : Gain  Gain=-1
  Gain1 : Gain  Gain=-1
  Product : Product  RndMeth=Zero
  Sum of Elements : Sum  Inputs=+  OutScaling=2^-10
  Out1 : Outport
  wires:
  Gain/1 -> Bias/1
  Sum of Elements/1 -> Gain/1
  Bias/1 -> Compare To Zero/1, Gain1/1
  Gain1/1 -> Bias1/1
  Compare To Zero/1 -> Data Type Conversion3/1
  Bias1/1 -> Product/2
  Data Type Conversion3/1 -> Product/1
  Product/1 -> Out1/1
  In1/1 -> Sum of Elements/1

== system soft_radio/Frame Synch/Preamble XCorr/Correlator ==
  In1 : Inport
  In2 : Inport  Orientation=up  Port=2
  Abs1 : Abs  SampleTime=-1  SaturateOnIntegerOverflow=off
  Product : Product  RndMeth=Zero
  Sum of Elements : Sum  Inputs=+  OutScaling=2^-10
  Out1 : Outport
  wires:
  Product/1 -> Sum of Elements/1
  Sum of Elements/1 -> Abs1/1
  In2/1 -> Product/2
  In1/1 -> Product/1
  Abs1/1 -> Out1/1

== system soft_radio/Frame Synch/Pulse On Preamble End/Latch high ==
  In1 : Inport
  Logical Operator2 : Logic  Operator=OR  AllPortsSameDT=off  OutDataTypeMode=Boolean
  Unit Delay : UnitDelay  Orientation=left  SampleTime=-1
  Out1 : Outport
  wires:
  Unit Delay/1 -> Logical Operator2/1
  Logical Operator2/1 -> Unit Delay/1, Out1/1
  In1/1 -> Logical Operator2/2

== system soft_radio/OFDM Demodulation/Carrier Synchronization and Channel Phase Comp/Angle1 ==
  In : Inport
  Complex to Magnitude-Angle : ComplexToMagnitudeAngle
  Terminator : Terminator
  Out : Outport
  wires:
  Complex to Magnitude-Angle/2 -> Out/1
  In/1 -> Complex to Magnitude-Angle/1
  Complex to Magnitude-Angle/1 -> Terminator/1
